simulink model "EMDTest"  (R2021b)
settings: Solver=VariableStepAuto  StartTime=0.0  StopTime=10.0  RelTol=1e-3
libraries: EMD x2
settings Model: Creator=Szalay  LastModifiedBy=Szalay

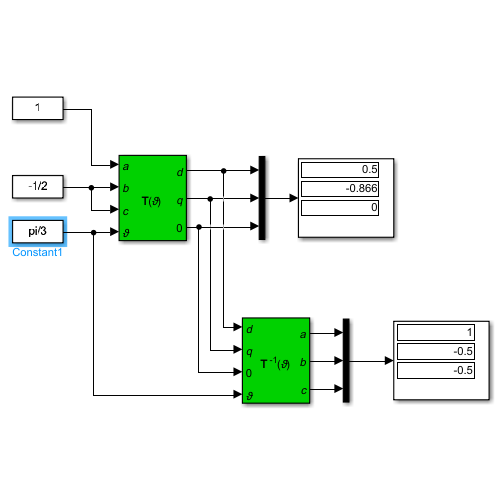
[thumbnail: Simulink's stored preview of the top-level diagram]
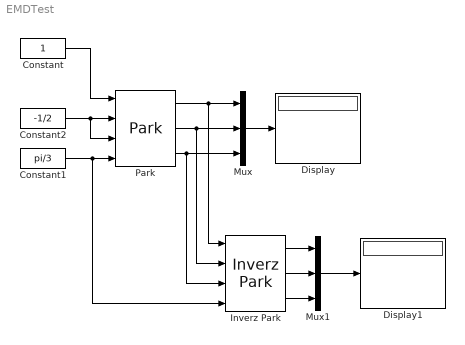
== system EMDTest ==
  Constant : Constant
  Constant1 : Constant  Value=pi/3
  Constant2 : Constant  Value=-1/2
  Display : Display
  Display1 : Display
  Inverz Park : EMD/Inverz Park  SystemSampleTime=-1  VariantActivationTime=update diagram  Latency=0  AutoFrameSizeCalculation=off
  Mux : Mux  Inputs=3
  Mux1 : Mux  Inputs=3
  Park : EMD/Park  SystemSampleTime=-1  VariantActivationTime=update diagram  Latency=0  AutoFrameSizeCalculation=off
  wires:
  Constant/1 -> Park/1
  Park/1 -> Inverz Park/1, Mux/1
  Park/2 -> Inverz Park/2, Mux/2
  Park/3 -> Inverz Park/3, Mux/3
  Mux/1 -> Display/1
  Constant1/1 -> Inverz Park/4, Park/4
  Constant2/1 -> Park/3, Park/2
  Mux1/1 -> Display1/1
  Inverz Park/3 -> Mux1/3
  Inverz Park/2 -> Mux1/2
  Inverz Park/1 -> Mux1/1
